simulink model "QPSK_mod_RasPi"  (R2019a)
settings: Solver=VariableStepAuto  StartTime=0.0  StopTime=inf  RelTol=1e-3
libraries: commfilt2 x2, dspsrcs4 x2, embdlinuxlib x1, commrandsrc3 x1, commdigbbndpm3 x1
settings Model: Creator=dom  LastModifiedBy=dom

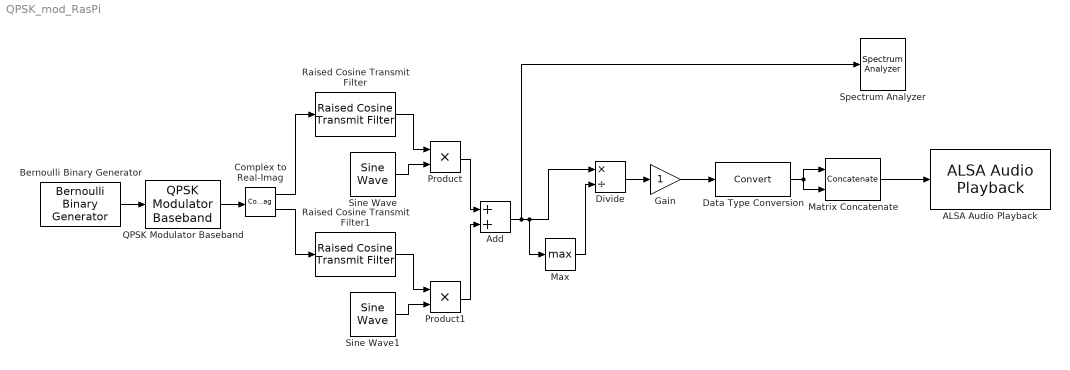
== system QPSK_mod_RasPi ==
  ALSA Audio Playback : embdlinuxlib/ALSA Audio Playback  deviceStr='plughw:0,0'  sampleRateEnum=48e3  queueDuration=0.5  blockPlatform=Raspberry Pi
      settings: SourceProductName=Simulink Coder Support Package for BeagleBone Blue Hardware  SourceProductBaseCode=SC_BEAGLEBONE_BLUE
  Add : Sum
  Bernoulli Binary Generator : commrandsrc3/Bernoulli Binary Generator  ProbabilityOfZero=0.5  SeedSource=Parameter  Seed=61  SampleTime=20/(2*48e3)  SamplesPerFrame=200  OutputDataType=double  SimulateUsing=Interpreted execution
      settings: SourceProductName=Communications Toolbox
  Complex to Real-Imag : ComplexToRealImag
  Data Type Conversion : DataTypeConversion
  Divide : Product  Inputs=*/
  Gain : Gain
  Matrix Concatenate : Concatenate  Mode=Multidimensional array  ConcatenateDimension=2
  Max : MinMax  Function=max
  Product : Product
  Product1 : Product
  QPSK Modulator Baseband : commdigbbndpm3/QPSK Modulator Baseband  InType=Bit  Enc=Binary  Ph=pi/4  outDtype=double  outWordLen=16  outUDDataType=sfix(16)  outFracLenMode=Best precision  outFracLen=15  outDataTypeStr=double  outLastDataTypeStr=double
      settings: SourceProductName=Communications Toolbox
  Raised Cosine Transmit Filter : commfilt2/Raised Cosine Transmit Filter  filtType=Square root  R=0.8  filtSpan=10  N=20  filterGain=1  InputProcessing=Columns as channels (frame based)  RateOptions=Enforce single-rate processing  framing=Mute  checkCoeff=off  variableName=rcTxFilt  checkGain=Normalized  sampMode=Mute  saveAsFlag=0  currentFiltSpan=10  D=5  launchFVT=on  roundingMode=Floor  overflowMode=off  coeffDataTypeStr=Inherit: Same word length as input  coeffMin=[]  coeffMax=[]  coeffLastDataTypeStr=Inherit: Same word length as input  outputDataTypeStr=Inherit: Same as accumulator  outputMin=[]  outputMax=[]  outputLastDataTypeStr=Inherit: Same as accumulator
      settings: SourceProductName=Communications Toolbox
  Raised Cosine Transmit Filter1 : commfilt2/Raised Cosine Transmit Filter  filtType=Square root  R=0.8  filtSpan=10  N=20  filterGain=1  InputProcessing=Columns as channels (frame based)  RateOptions=Enforce single-rate processing  framing=Mute  checkCoeff=off  variableName=rcTxFilt1  checkGain=Normalized  sampMode=Mute  saveAsFlag=0  currentFiltSpan=10  D=5  launchFVT=on  roundingMode=Floor  overflowMode=off  coeffDataTypeStr=Inherit: Same word length as input  coeffMin=[]  coeffMax=[]  coeffLastDataTypeStr=Inherit: Same word length as input  outputDataTypeStr=Inherit: Same as accumulator  outputMin=[]  outputMax=[]  outputLastDataTypeStr=Inherit: Same as accumulator
      settings: SourceProductName=Communications Toolbox
  Sine Wave : dspsrcs4/Sine Wave  Amplitude=1  Frequency=15e3  Phase=pi/2  SampleMode=Discrete  OutComplex=Real  CompMethod=Trigonometric fcn  TableSize=Speed  SampleTime=1/48e3  SamplesPerFrame=2e3  ResetState=Restart at time zero  OutputFrames=off  dataType=double  wordLen=16  udDataType=sfix(16)  fracBitsMode=Best precision  numFracBits=15  OutDataTypeStr=double  LastOutDataTypeStr=double
  Sine Wave1 : dspsrcs4/Sine Wave  Amplitude=1  Frequency=15e3  Phase=pi  SampleMode=Discrete  OutComplex=Real  CompMethod=Trigonometric fcn  TableSize=Speed  SampleTime=1/48e3  SamplesPerFrame=2e3  ResetState=Restart at time zero  OutputFrames=off  dataType=double  wordLen=16  udDataType=sfix(16)  fracBitsMode=Best precision  numFracBits=15  OutDataTypeStr=double  LastOutDataTypeStr=double
  Spectrum Analyzer : SpectrumAnalyzer
  wires:
  Bernoulli Binary Generator/1 -> QPSK Modulator Baseband/1
  QPSK Modulator Baseband/1 -> Complex to Real-Imag/1
  Complex to Real-Imag/1 -> Raised Cosine Transmit Filter/1
  Sine Wave/1 -> Product/2
  Raised Cosine Transmit Filter/1 -> Product/1
  Product/1 -> Add/1
  Divide/1 -> Gain/1
  Matrix Concatenate/1 -> ALSA Audio Playback/1
  Gain/1 -> Data Type Conversion/1
  Data Type Conversion/1 -> Matrix Concatenate/2, Matrix Concatenate/1
  Product1/1 -> Add/2
  Raised Cosine Transmit Filter1/1 -> Product1/1
  Sine Wave1/1 -> Product1/2
  Complex to Real-Imag/2 -> Raised Cosine Transmit Filter1/1
  Add/1 -> Spectrum Analyzer/1, Max/1, Divide/1
  Max/1 -> Divide/2
